simulink model "Final_FCcontrol"  (R2023a)
settings: Solver=VariableStepAuto  StartTime=0.0  StopTime=22  RelTol=1e-3
values from neighbouring files (symbols this model uses):
  I_P_TLU =     [current_pressure_TLU.mat]
undefined symbols (not defined in the file or in its folder): A_cell, N_cell
settings Model: Creator=Abhinandan  LastModifiedBy=Abhinandan

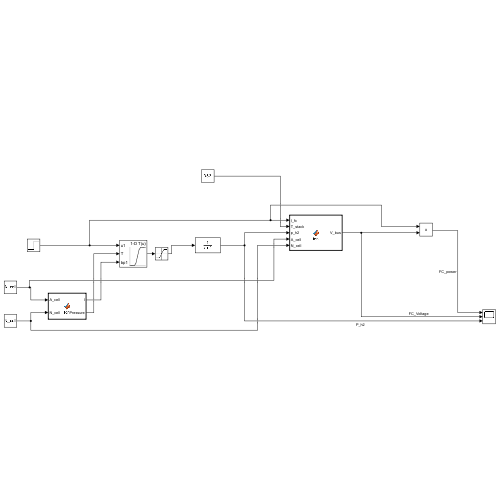
[thumbnail: Simulink's stored preview of the top-level diagram]
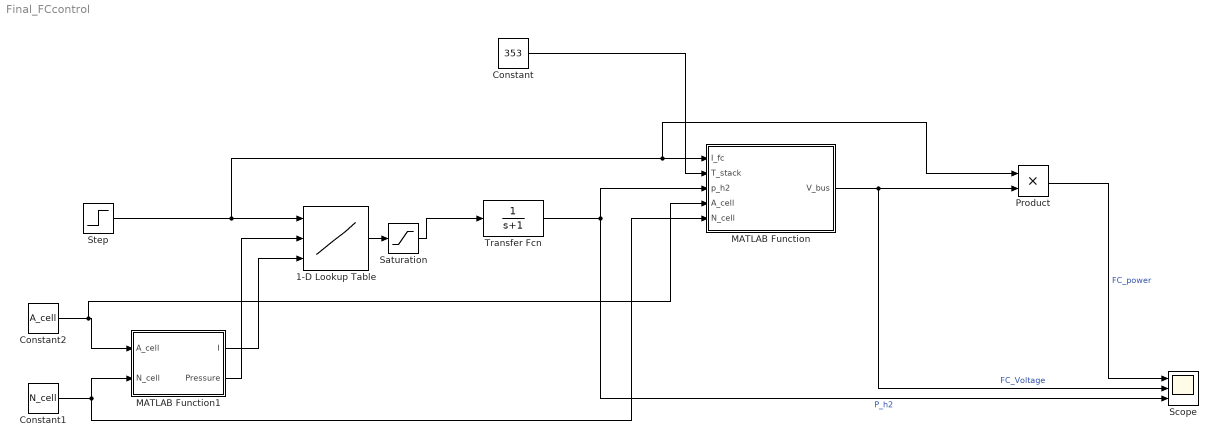
== system Final_FCcontrol ==
  1-D Lookup Table : Lookup_n-D  NumberOfTableDimensions=1  BreakpointsForDimension1Source=Input port  BreakpointsForDimension1=I_P_TLU.Current  TableSource=Input port  Table=I_P_TLU.Pressure  InternalRulePriority=Speed  RndMeth=Simplest
      settings: InputPortMap=u0,p221,p5
  Constant : Constant  Value=353
  Constant1 : Constant  Value=N_cell
  Constant2 : Constant  Value=A_cell
  MATLAB Function : MATLAB Function  TreatAsAtomicUnit=on
  MATLAB Function1 : MATLAB Function  TreatAsAtomicUnit=on
  Product : Product
  Saturation : Saturate  UpperLimit=1.5  LowerLimit=0
  Scope : Scope  NumInputPorts=3
  Step : Step  Time=15  Before=107  After=154  SampleTime=0
  Transfer Fcn : TransferFcn  Denominator=[1 1]
  wires:
  1-D Lookup Table/1 -> Saturation/1
  Transfer Fcn/1 -> Scope/3, MATLAB Function/3(p_h2)  "P_h2"
  Constant/1 -> MATLAB Function/2(T_stack)
  MATLAB Function/1(V_bus) -> Scope/2, Product/2  "FC_Voltage"
  Product/1 -> Scope/1  "FC_power"
  Step/1 -> Product/1, MATLAB Function/1(I_fc), 1-D Lookup Table/1
  MATLAB Function1/1(I) -> 1-D Lookup Table/3
  MATLAB Function1/2(Pressure) -> 1-D Lookup Table/2
  Constant1/1 -> MATLAB Function/5(N_cell), MATLAB Function1/2(N_cell)
  Constant2/1 -> MATLAB Function/4(A_cell), MATLAB Function1/1(A_cell)
  Saturation/1 -> Transfer Fcn/1

== matlab function Final_FCcontrol/MATLAB Function1 ==
  data: A_cell input; I output; Pressure output; N_cell input
function [I,Pressure] = fcn(A_cell,N_cell)

    P_range = linspace(0.1,1.5);
    I_range = linspace(0,450,10000);
    I = zeros(100,1);
    Pressure = zeros(100,1);
    for j = 1:size(P_range,2)
        for i = 1:size(I_range,2)
            V = fcn(P_range(1,j),I_range(1,i),353);
            if (V>246 && V<254)
                I(j,1) = I_range(1,i);
                Pressure(j,1) = P_range(1,j);
            end
        end
    end
    
    
    function V_bus = fcn(p_h2,I_fc,T_stack)                %T_stack in K, T_fc in A, V_bus in V
        F = 96485.33;       
        R = 8.31447;
        i_lim = 1.4;
    
        E_cell = -237.14e+3/(-2*F);
        i_cell = I_fc/A_cell;
        
        i0 = 8e-05;
        alpha = 0.5;
        t_membrane = 125e-4;
        
        a = 0.5;
        lambda_m = 0.043 + 17.81*a - 39.85*a^2 + 36*a^3;
        sigma_30 = 0.005139*lambda_m - 0.00326;
        sigma = sigma_30*exp(1268*(1/303.15 - 1/T_stack));
        
        b = (R*T_stack)/(2*alpha*F);  
    
        V_nernst = E_cell + R*T_stack/(2*F) * log((3/4)^(1/2)*p_h2^(3/2));
    
        V_act = b*log(i_cell/i0);
    
        R_ohm = t_membrane/sigma;
        V_ohm = i_cell*R_ohm;
    
        V_conc = -R*T_stack/(2*F) * log(1-(i_cell/i_lim));          
        V_cell = V_nernst - V_act - V_ohm - V_conc;
    
    
        V_bus = V_cell*N_cell;
    end
end

== matlab function Final_FCcontrol/MATLAB Function ==
  data: I_fc input; T_stack input; p_h2 input; V_bus output; A_cell input; N_cell input
function V_bus = fcn(I_fc,T_stack,p_h2,A_cell,N_cell)                %T_stack in K, T_fc in A, V_bus in V
    F = 96485.33;       
    R = 8.31447;
    i_lim = 1.4;

    E_cell = -237.14e+3/(-2*F);
    i_cell = I_fc/A_cell;
    
    i0 = 8e-05;
    alpha = 0.5;
    t_membrane = 125e-4;
    
    a = 0.5;
    lambda_m = 0.043 + 17.81*a - 39.85*a^2 + 36*a^3;
    sigma_30 = 0.005139*lambda_m - 0.00326;
    sigma = sigma_30*exp(1268*(1/303.15 - 1/T_stack));
    
    b = (R*T_stack)/(2*alpha*F);  

    V_nernst = E_cell + R*T_stack/(2*F) * log((3/4)^(1/2)*p_h2^(3/2));

    V_act = b*log(i_cell/i0);

    R_ohm = t_membrane/sigma;
    V_ohm = i_cell*R_ohm;

    V_conc = -R*T_stack/(2*F) * log(1-(i_cell/i_lim));          
    V_cell = V_nernst - V_act - V_ohm - V_conc;


    V_bus = V_cell*N_cell;
end
